simulink model "PMSM_simul"  (R2021a)
settings: Solver=VariableStepAuto  StartTime=0.0  StopTime=0.5  RelTol=1e-3
values from neighbouring files (symbols this model uses):
  Bm = 0.0001    [PMSM.m]
  I_max = 100    [PMSM.m]
  Jm = 0.00015    [PMSM.m]
  kacd = 1/kpcd    (= 0.010301290815)    [PMSM.m]
  kacq = 1/kpcq    (= 0.0058191935317)    [PMSM.m]
  kas = 1/kps    (= 47.7464829276)    [PMSM.m]
  kicd = Rs*wcc    (= 13823.0076758)    [PMSM.m]
  kicq = Rs*wcc    (= 13823.0076758)    [PMSM.m]
  kis = kps*wcs/5    (= 13.1594725348)    [PMSM.m]
  kpcd = Ld*wcc    (= 97.0752129959)    [PMSM.m]
  kpcq = Lq*wcc    (= 171.845118151)    [PMSM.m]
  kps = Jm*wcs/Kt    (= 0.0209439510239)    [PMSM.m]
  LAMpm = 0.0976    [PMSM.m]
  Ld = 3.09*10^-3    (= 0.00309)    [PMSM.m]
  Lq = 5.47*10^-3    (= 0.00547)    [PMSM.m]
  Pol = 6    [PMSM.m]
  Rs = 0.44    [PMSM.m]
  V_max = 212    [PMSM.m]
  Wrpmref = 1000    [PMSM.m]
settings Model: Creator=syl12  LastModifiedBy=syl12

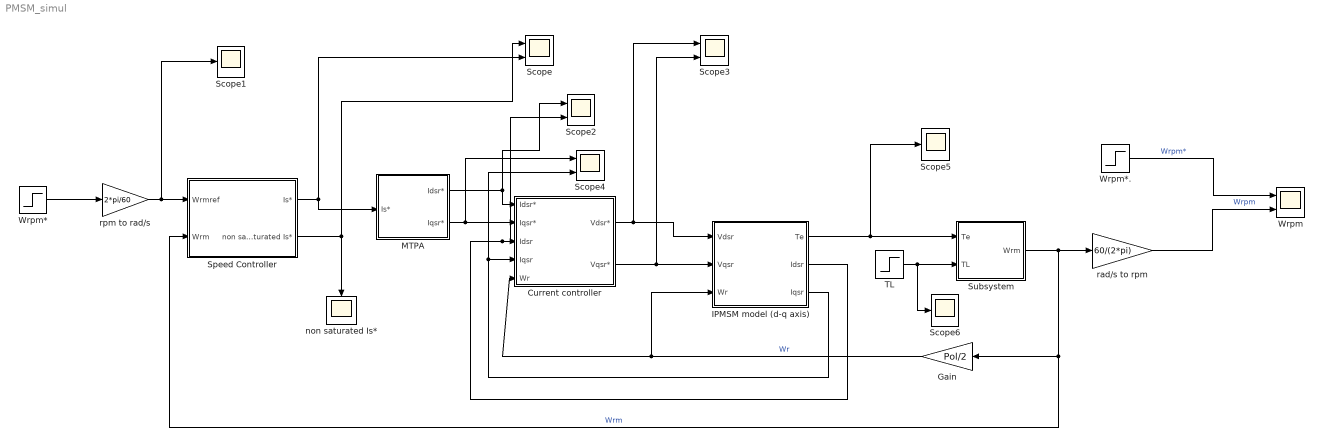
== system PMSM_simul ==
  Current controller : Subsystem
  Gain : Gain  Gain=Pol/2
  IPMSM model (d-q axis) : Subsystem
  MTPA : Subsystem
  Scope{,2..4} (4 alike) : Scope  NumInputPorts=2
  Scope1 : Scope
  Scope5 : Scope
  Scope6 : Scope
  Speed Controller : Subsystem
  Subsystem : Subsystem
  TL : Step  Time=0.3  Before=3  After=4  SampleTime=0
  Wrpm : Scope  NumInputPorts=2
  Wrpm* : Step  Time=0  After=Wrpmref  SampleTime=0
  Wrpm*. : Step  Time=0  After=Wrpmref  SampleTime=0
  non saturated Is* : Scope
  "rad/s to rpm  " : Gain  Gain=60/(2*pi)
  rpm to rad/s : Gain  Gain=2*pi/60
  wires:
  Wrpm*/1 -> rpm to rad/s/1
  rpm to rad/s/1 -> Scope1/1, Speed Controller/1(Wrmref)
  Speed Controller/1(Is*) -> Scope/2, MTPA/1(Is*)
  Speed Controller/2(non saturated Is*) -> Scope/1, non saturated Is*/1
  MTPA/1(Idsr*) -> Current controller/1(Idsr*), Scope2/1
  MTPA/2(Iqsr*) -> Current controller/2(Iqsr*), Scope4/1
  Current controller/1(Vdsr*) -> Scope3/1, IPMSM model (d-q axis)/1(Vdsr)
  Current controller/2(Vqsr*) -> Scope3/2, IPMSM model (d-q axis)/2(Vqsr)
  IPMSM model (d-q axis)/2(Idsr) -> Scope2/2, Current controller/3(Idsr)
  IPMSM model (d-q axis)/3(Iqsr) -> Scope4/2, Current controller/4(Iqsr)
  IPMSM model (d-q axis)/1(Te) -> Scope5/1, Subsystem/1(Te)
  TL/1 -> Scope6/1, Subsystem/2(TL)
  Subsystem/1(Wrm) -> Speed Controller/2(Wrm), Gain/1, "rad/s to rpm  "/1  "Wrm"
  "rad/s to rpm  "/1 -> Wrpm/2  "Wrpm"
  Gain/1 -> IPMSM model (d-q axis)/3(Wr), Current controller/5(Wr)  "Wr"
  Wrpm*./1 -> Wrpm/1  "Wrpm*"

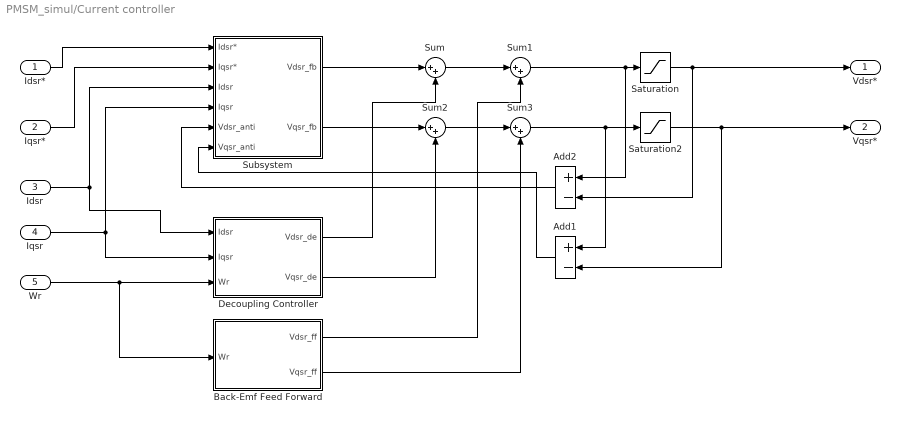
== system PMSM_simul/Current controller ==
  Idsr* : Inport
  Iqsr* : Inport  Port=2
  Idsr : Inport  Port=3
  Iqsr : Inport  Port=4
  Wr : Inport  Port=5
  Add1 : Sum  Inputs=+-
  Add2 : Sum  Inputs=+-
  Back-Emf Feed Forward : Subsystem
  Decoupling Controller : Subsystem
  Saturation : Saturate  UpperLimit=V_max  LowerLimit=-V_max
  Saturation2 : Saturate  UpperLimit=V_max  LowerLimit=-V_max
  Subsystem : Subsystem
  Sum{,1..3} (4 alike) : Sum  Inputs=|++
  Vdsr* : Outport
  Vqsr* : Outport  Port=2
  wires:
  Sum/1 -> Sum1/1
  Sum2/1 -> Sum3/1
  Sum1/1 -> Add2/1, Saturation/1
  Decoupling Controller/1(Vdsr_de) -> Sum/2
  Saturation/1 -> Add2/2, Vdsr*/1
  Sum3/1 -> Saturation2/1, Add1/1
  Back-Emf Feed Forward/1(Vdsr_ff) -> Sum1/2
  Decoupling Controller/2(Vqsr_de) -> Sum2/2
  Back-Emf Feed Forward/2(Vqsr_ff) -> Sum3/2
  Wr/1 -> Decoupling Controller/3(Wr), Back-Emf Feed Forward/1(Wr)
  Subsystem/1(Vdsr_fb) -> Sum/1
  Subsystem/2(Vqsr_fb) -> Sum2/1
  Idsr*/1 -> Subsystem/1(Idsr*)
  Iqsr*/1 -> Subsystem/2(Iqsr*)
  Idsr/1 -> Decoupling Controller/1(Idsr), Subsystem/3(Idsr)
  Iqsr/1 -> Decoupling Controller/2(Iqsr), Subsystem/4(Iqsr)
  Saturation2/1 -> Add1/2, Vqsr*/1
  Add2/1 -> Subsystem/5(Vdsr_anti)
  Add1/1 -> Subsystem/6(Vqsr_anti)

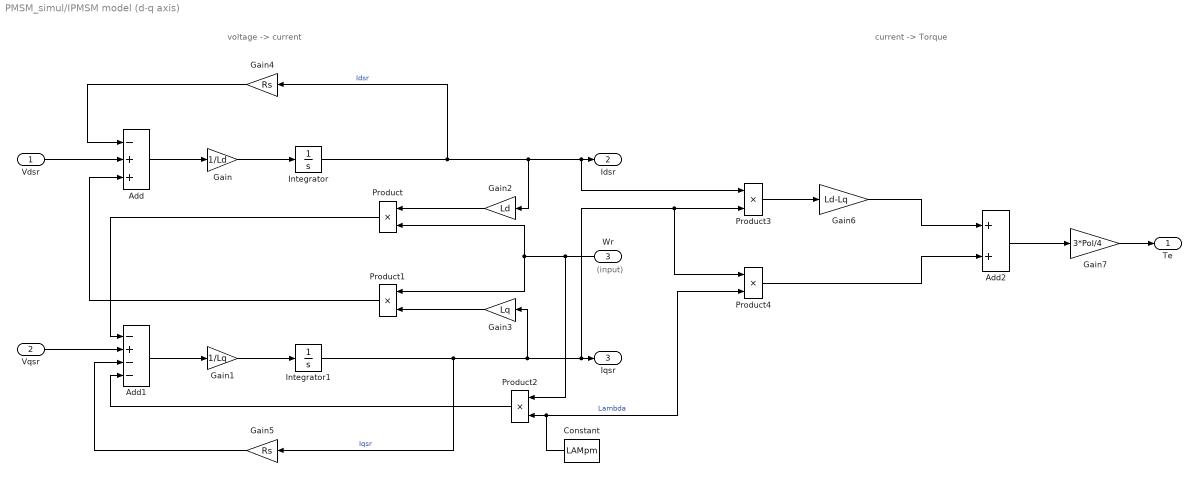
== system PMSM_simul/IPMSM model (d-q axis) ==
  note: voltage -> current
  note: (input)
  note: current -> Torque
  Vdsr : Inport
  Vqsr : Inport  Port=2
  Wr : Inport  Port=3
  Add : Sum  Inputs=-++
  Add1 : Sum  Inputs=-+--
  Add2 : Sum
  Constant : Constant  Value=LAMpm
  Gain : Gain  Gain=1/Ld
  Gain1 : Gain  Gain=1/Lq
  Gain2 : Gain  Gain=Ld
  Gain3 : Gain  Gain=Lq
  Gain4 : Gain  Gain=Rs
  Gain5 : Gain  Gain=Rs
  Gain6 : Gain  Gain=Ld-Lq
  Gain7 : Gain  Gain=3*Pol/4
  Integrator : Integrator
  Integrator1 : Integrator
  Product{,1..4} (5 alike) : Product
  Te : Outport
  Idsr : Outport  Port=2
  Iqsr : Outport  Port=3
  wires:
  Vdsr/1 -> Add/2
  Add/1 -> Gain/1
  Gain/1 -> Integrator/1
  Integrator/1 -> Gain4/1, Gain2/1, Product3/1, Idsr/1  "Idsr"
  Gain4/1 -> Add/1
  Vqsr/1 -> Add1/2
  Gain1/1 -> Integrator1/1
  Add1/1 -> Gain1/1
  Integrator1/1 -> Gain5/1, Gain3/1, Product3/2, Product4/1, Iqsr/1  "Iqsr"
  Gain3/1 -> Product1/2
  Gain2/1 -> Product/1
  Wr/1 -> Product1/1, Product/2, Product2/1
  Product/1 -> Add1/1
  Product1/1 -> Add/3
  Gain5/1 -> Add1/3
  Constant/1 -> Product4/2, Product2/2  "Lambda"
  Product2/1 -> Add1/4
  Product3/1 -> Gain6/1
  Gain6/1 -> Add2/1
  Product4/1 -> Add2/2
  Add2/1 -> Gain7/1
  Gain7/1 -> Te/1

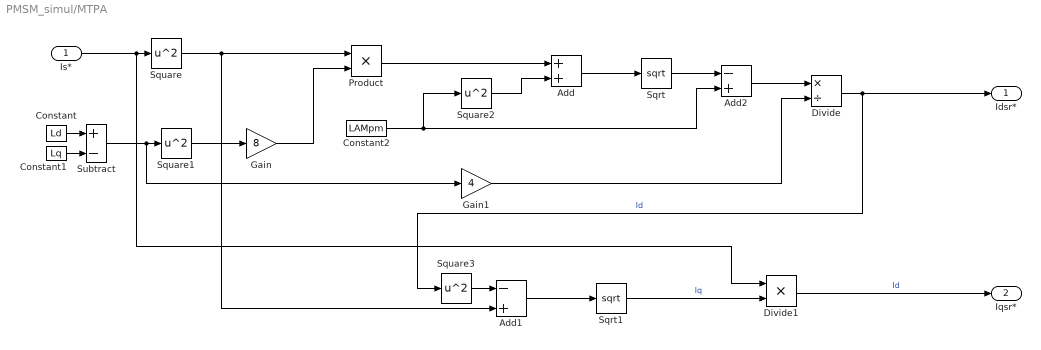
== system PMSM_simul/MTPA ==
  Is* : Inport
  Add : Sum
  Add1 : Sum  Inputs=-+
  Add2 : Sum  Inputs=-+
  Constant : Constant  Value=Ld
  Constant1 : Constant  Value=Lq
  Constant2 : Constant  Value=LAMpm
  Divide : Product  Inputs=*/
  Divide1 : Product  Inputs=**
  Gain : Gain  Gain=8
  Gain1 : Gain  Gain=4
  Product : Product
  Sqrt : Sqrt  SaturateOnIntegerOverflow=on
  Sqrt1 : Sqrt  SaturateOnIntegerOverflow=on
  Square{,1..3} (4 alike) : Math  Operator=square  SaturateOnIntegerOverflow=on
  Subtract : Sum  Inputs=+-
  Idsr* : Outport
  Iqsr* : Outport  Port=2
  wires:
  Constant/1 -> Subtract/1
  Constant1/1 -> Subtract/2
  Is*/1 -> Divide1/1, Square/1
  Square/1 -> Product/1, Add1/2
  Subtract/1 -> Gain1/1, Square1/1
  Square1/1 -> Gain/1
  Gain/1 -> Product/2
  Product/1 -> Add/1
  Constant2/1 -> Add2/2, Square2/1
  Square2/1 -> Add/2
  Add/1 -> Sqrt/1
  Sqrt/1 -> Add2/1
  Add2/1 -> Divide/1
  Gain1/1 -> Divide/2
  Divide/1 -> Square3/1, Idsr*/1  "Id"
  Add1/1 -> Sqrt1/1
  Square3/1 -> Add1/1
  Sqrt1/1 -> Divide1/2  "Iq"
  Divide1/1 -> Iqsr*/1  "Id"

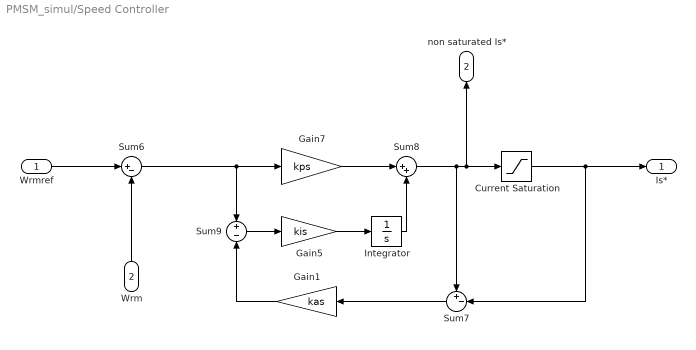
== system PMSM_simul/Speed Controller ==
  Wrmref : Inport
  Wrm : Inport  Port=2
  Current Saturation : Saturate  UpperLimit=I_max  LowerLimit=-I_max  ZeroCross=off
  Gain1 : Gain  Gain=kas
  Gain5 : Gain  Gain=kis
  Gain7 : Gain  Gain=kps
  Integrator : Integrator
  Sum6 : Sum  Inputs=|+-
  Sum7 : Sum  Inputs=+-|
  Sum8 : Sum  Inputs=|++
  Sum9 : Sum  Inputs=+|-
  Is* : Outport
  non saturated Is* : Outport  Port=2
  wires:
  Sum9/1 -> Gain5/1
  Wrmref/1 -> Sum6/1
  Gain7/1 -> Sum8/1
  Sum7/1 -> Gain1/1
  Sum6/1 -> Sum9/1, Gain7/1
  Integrator/1 -> Sum8/2
  Gain1/1 -> Sum9/2
  Wrm/1 -> Sum6/2
  Current Saturation/1 -> Is*/1, Sum7/2
  Sum8/1 -> Sum7/1, non saturated Is*/1, Current Saturation/1
  Gain5/1 -> Integrator/1

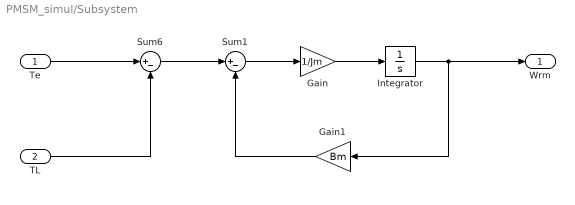
== system PMSM_simul/Subsystem ==
  Te : Inport
  TL : Inport  Port=2
  Gain : Gain  Gain=1/Jm
  Gain1 : Gain  Gain=Bm
  Integrator : Integrator
  Sum1 : Sum  Inputs=|+-
  Sum6 : Sum  Inputs=|+-
  Wrm : Outport
  wires:
  Te/1 -> Sum6/1
  TL/1 -> Sum6/2
  Sum6/1 -> Sum1/1
  Integrator/1 -> Gain1/1, Wrm/1
  Gain1/1 -> Sum1/2
  Sum1/1 -> Gain/1
  Gain/1 -> Integrator/1

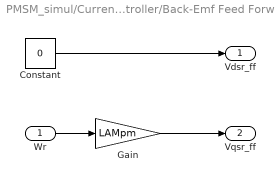
== system PMSM_simul/Current controller/Back-Emf Feed Forward ==
  Wr : Inport
  Constant : Constant  Value=0
  Gain : Gain  Gain=LAMpm
  Vdsr_ff : Outport
  Vqsr_ff : Outport  Port=2
  wires:
  Constant/1 -> Vdsr_ff/1
  Gain/1 -> Vqsr_ff/1
  Wr/1 -> Gain/1

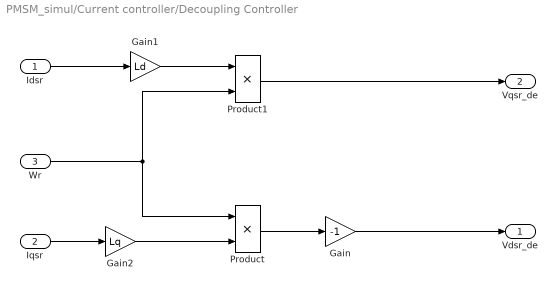
== system PMSM_simul/Current controller/Decoupling Controller ==
  Idsr : Inport
  Iqsr : Inport  Port=2
  Wr : Inport  Port=3
  Gain : Gain  Gain=-1
  Gain1 : Gain  Gain=Ld
  Gain2 : Gain  Gain=Lq
  Product : Product
  Product1 : Product
  Vdsr_de : Outport
  Vqsr_de : Outport  Port=2
  wires:
  Idsr/1 -> Gain1/1
  Gain1/1 -> Product1/1
  Wr/1 -> Product/1, Product1/2
  Iqsr/1 -> Gain2/1
  Gain2/1 -> Product/2
  Product/1 -> Gain/1
  Product1/1 -> Vqsr_de/1
  Gain/1 -> Vdsr_de/1

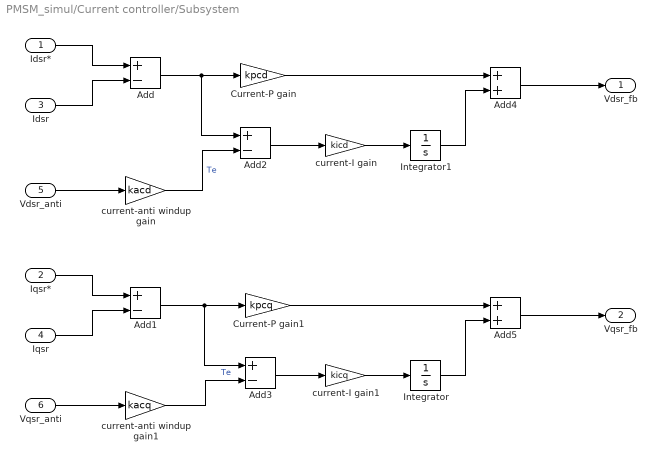
== system PMSM_simul/Current controller/Subsystem ==
  Idsr* : Inport
  Iqsr* : Inport  Port=2
  Idsr : Inport  Port=3
  Iqsr : Inport  Port=4
  Vdsr_anti : Inport  Port=5
  Vqsr_anti : Inport  Port=6
  Add{,1..3} (4 alike) : Sum  Inputs=+-
  Add4 : Sum
  Add5 : Sum
  Current-P gain : Gain  Gain=kpcd
  Current-P gain1 : Gain  Gain=kpcq
  Integrator : Integrator
  Integrator1 : Integrator
  current-I gain : Gain  Gain=kicd
  current-I gain1 : Gain  Gain=kicq
  current-anti windup gain : Gain  Gain=kacd
  current-anti windup gain1 : Gain  Gain=kacq
  Vdsr_fb : Outport
  Vqsr_fb : Outport  Port=2
  wires:
  Vqsr_anti/1 -> current-anti windup gain1/1
  Vdsr_anti/1 -> current-anti windup gain/1
  Idsr*/1 -> Add/1
  Idsr/1 -> Add/2
  Iqsr*/1 -> Add1/1
  Iqsr/1 -> Add1/2
  current-anti windup gain1/1 -> Add3/2  "Te"
  Add1/1 -> Add3/1, Current-P gain1/1
  current-anti windup gain/1 -> Add2/2  "Te"
  Add/1 -> Add2/1, Current-P gain/1
  Add5/1 -> Vqsr_fb/1
  Add4/1 -> Vdsr_fb/1
  Add3/1 -> current-I gain1/1
  Add2/1 -> current-I gain/1
  current-I gain1/1 -> Integrator/1
  current-I gain/1 -> Integrator1/1
  Current-P gain1/1 -> Add5/1
  Current-P gain/1 -> Add4/1
  Integrator1/1 -> Add4/2
  Integrator/1 -> Add5/2
